simulink model "ProMesh_DualBand_BaseStation"  (R2024b)
settings: Solver=FixedStepAuto  StartTime=0.0  StopTime=210  FixedStep=1  RelTol=1e-3
settings Model: Creator=ARYA MGC  LastModifiedBy=ARYA MGC

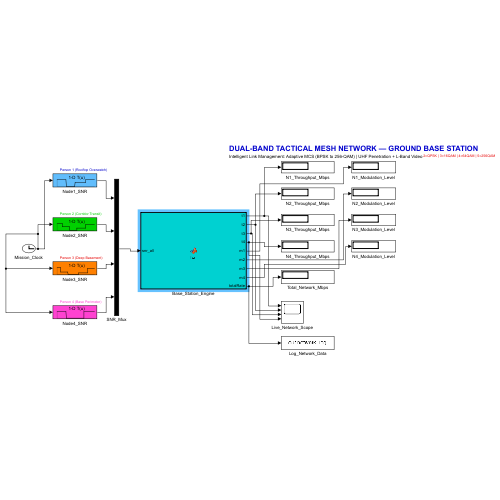
[thumbnail: Simulink's stored preview of the top-level diagram]
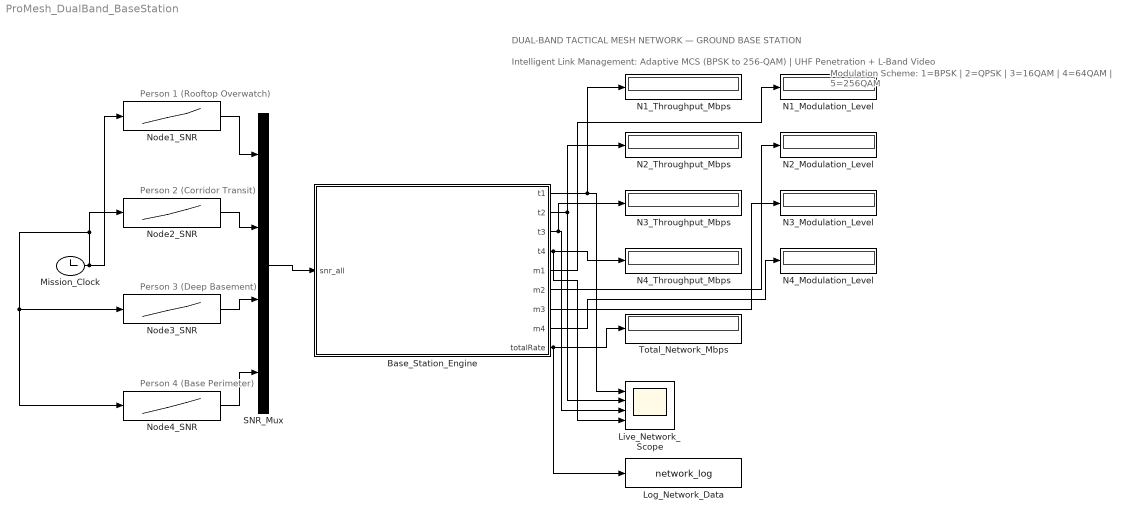
== system ProMesh_DualBand_BaseStation ==
  note: DUAL-BAND TACTICAL MESH NETWORK — GROUND BASE STATION
  note: Intelligent Link Management: Adaptive MCS (BPSK to 256-QAM) | UHF Penetration + L-Band Video
  note: Person 1 (Rooftop Overwatch)
  note: Person 2 (Corridor Transit)
  note: Person 3 (Deep Basement)
  note: Person 4 (Base Perimeter)
  note: Modulation Scheme: 1=BPSK | 2=QPSK | 3=16QAM | 4=64QAM | 5=256QAM
  Base_Station_Engine : MATLAB Function  TreatAsAtomicUnit=on
  Live_Network_Scope : Scope  NumInputPorts=4
  Log_Network_Data : ToWorkspace  VariableName=network_log  SampleTime=-1
  Mission_Clock : Clock
  N1_Modulation_Level : Display
  N1_Throughput_Mbps : Display
  N2_Modulation_Level : Display
  N2_Throughput_Mbps : Display
  N3_Modulation_Level : Display
  N3_Throughput_Mbps : Display
  N4_Modulation_Level : Display
  N4_Throughput_Mbps : Display
  Node1_SNR : Lookup_n-D  NumberOfTableDimensions=1  BreakpointsForDimension1=[0 50 51 100 101 160 161 210]  Table=[30 30 18 18 25 25 30 30]  InternalRulePriority=Speed  RndMeth=Simplest
  Node2_SNR : Lookup_n-D  NumberOfTableDimensions=1  BreakpointsForDimension1=[0 30 31 70 71 110 111 160 161 210]  Table=[22 22 15 15 8 8 12 12 20 20]  InternalRulePriority=Speed  RndMeth=Simplest
  Node3_SNR : Lookup_n-D  NumberOfTableDimensions=1  BreakpointsForDimension1=[0 20 21 60 61 120 121 170 171 210]  Table=[20 20 10 10 5 5 8 8 18 18]  InternalRulePriority=Speed  RndMeth=Simplest
  Node4_SNR : Lookup_n-D  NumberOfTableDimensions=1  BreakpointsForDimension1=[0 50 51 150 151 210]  Table=[25 25 20 20 25 25]  InternalRulePriority=Speed  RndMeth=Simplest
  SNR_Mux : Mux
  Total_Network_Mbps : Display
  wires:
  Mission_Clock/1 -> Node4_SNR/1, Node3_SNR/1, Node2_SNR/1, Node1_SNR/1
  Node1_SNR/1 -> SNR_Mux/1
  Node2_SNR/1 -> SNR_Mux/2
  Node3_SNR/1 -> SNR_Mux/3
  Node4_SNR/1 -> SNR_Mux/4
  SNR_Mux/1 -> Base_Station_Engine/1(snr_all)
  Base_Station_Engine/1(t1) -> N1_Throughput_Mbps/1, Live_Network_Scope/1
  Base_Station_Engine/2(t2) -> N2_Throughput_Mbps/1, Live_Network_Scope/2
  Base_Station_Engine/3(t3) -> N3_Throughput_Mbps/1, Live_Network_Scope/3
  Base_Station_Engine/4(t4) -> N4_Throughput_Mbps/1, Live_Network_Scope/4
  Base_Station_Engine/5(m1) -> N1_Modulation_Level/1
  Base_Station_Engine/6(m2) -> N2_Modulation_Level/1
  Base_Station_Engine/7(m3) -> N3_Modulation_Level/1
  Base_Station_Engine/8(m4) -> N4_Modulation_Level/1
  Base_Station_Engine/9(totalRate) -> Total_Network_Mbps/1, Log_Network_Data/1

== matlab function ProMesh_DualBand_BaseStation/Base_Station_Engine ==
  data: snr_all input; t1 output; t2 output; t3 output; t4 output; m1 output; m2 output; m3 output; m4 output; totalRate output
function [t1, t2, t3, t4, m1, m2, m3, m4, totalRate] = fcn(snr_all)
coder.extrinsic('process_pro_mesh');
t1=0; t2=0; t3=0; t4=0; m1=1; m2=1; m3=1; m4=1; totalRate=0;
[t1, t2, t3, t4, m1, m2, m3, m4, totalRate] = process_pro_mesh(snr_all);
